simulink model "feedbackLin_Eq_Model"  (R2021a)
settings: Solver=ode1  StartTime=0.0  StopTime=150  FixedStep=0.005  RelTol=1e-3
undefined symbols (not defined in the file or in its folder): DiscIntNeverNeededParam
settings Model: Creator=laberobotica  LastModifiedBy=gabri

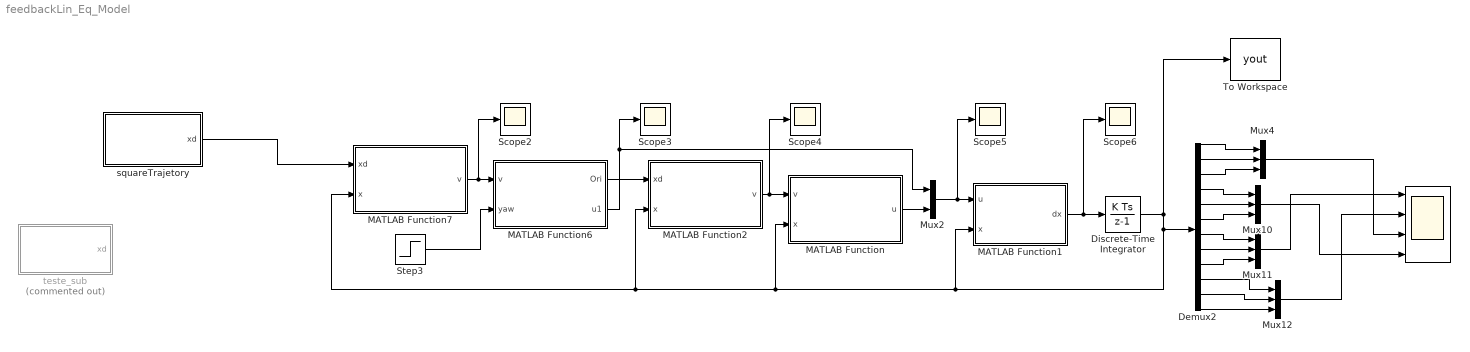
== system feedbackLin_Eq_Model ==
  " " : Scope  NumInputPorts=4
  Demux2 : Demux  Outputs=12
  Discrete-Time Integrator : DiscreteIntegrator  SampleTime=0.005  ICPrevOutput=DiscIntNeverNeededParam  ICPrevScaledInput=DiscIntNeverNeededParam
  MATLAB Function : MATLAB Function  TreatAsAtomicUnit=on
  MATLAB Function1 : MATLAB Function  TreatAsAtomicUnit=on
  MATLAB Function2 : MATLAB Function  TreatAsAtomicUnit=on
  MATLAB Function6 : MATLAB Function  TreatAsAtomicUnit=on
  MATLAB Function7 : MATLAB Function  TreatAsAtomicUnit=on
  Mux{4,10..12} (4 alike) : Mux  Inputs=3
  Mux2 : Mux  Inputs=2
  Scope{2..6} (5 alike) : Scope
  Step3 : Step  Time=35  After=0  SampleTime=0.005
  To Workspace : ToWorkspace  VariableName=yout  SampleTime=-1
      settings: Save2DSignal=2-D array (concatenate along first dimension)
  squareTrajetory : Subsystem
  teste_sub : Subsystem  Commented=on
  wires:
  MATLAB Function2/1(v) -> Scope4/1, MATLAB Function/1(v)
  MATLAB Function7/1(v) -> MATLAB Function6/1(v), Scope2/1
  Demux2/7 -> Mux11/1
  Demux2/9 -> Mux11/3
  Demux2/2 -> Mux4/2
  Demux2/10 -> Mux12/1
  Mux11/1 -> " "/1
  Mux4/1 -> " "/3
  Demux2/8 -> Mux11/2
  Discrete-Time Integrator/1 -> To Workspace/1, MATLAB Function1/2(x), MATLAB Function7/2(x), MATLAB Function2/2(x), MATLAB Function/2(x), Demux2/1
  Mux10/1 -> " "/4
  Mux12/1 -> " "/2
  Demux2/3 -> Mux4/3
  Demux2/11 -> Mux12/2
  Demux2/6 -> Mux10/3
  Demux2/12 -> Mux12/3
  Demux2/4 -> Mux10/1
  Demux2/5 -> Mux10/2
  Demux2/1 -> Mux4/1
  MATLAB Function6/2(u1) -> Mux2/1, Scope3/1
  MATLAB Function6/1(Ori) -> MATLAB Function2/1(xd)
  Step3/1 -> MATLAB Function6/2(yaw)
  MATLAB Function/1(u) -> Mux2/2
  Mux2/1 -> Scope5/1, MATLAB Function1/1(u)
  MATLAB Function1/1(dx) -> Discrete-Time Integrator/1, Scope6/1
  squareTrajetory/1(xd) -> MATLAB Function7/1(xd)

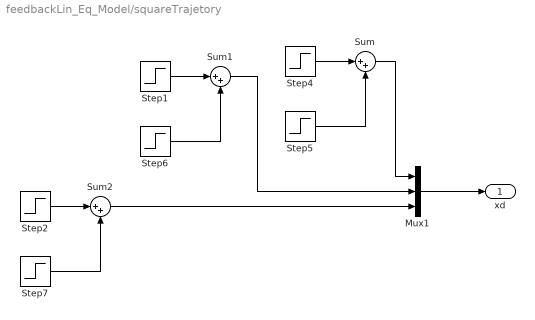
== system feedbackLin_Eq_Model/squareTrajetory ==
  Mux1 : Mux  Inputs=3
  Step1 : Step  Time=50  SampleTime=0.005
  Step2 : Step  Time=0  After=1.1  SampleTime=0.005
  Step4 : Step  Time=25  SampleTime=0.005
  Step5 : Step  Time=75  After=-1  SampleTime=0.005
  Step6 : Step  Time=100  After=-1  SampleTime=0.005
  Step7 : Step  Time=120  After=-1.1  SampleTime=0.005
  Sum : Sum  Inputs=|++
  Sum1 : Sum  Inputs=|++
  Sum2 : Sum  Inputs=|++
  xd : Outport
  wires:
  Step4/1 -> Sum/1
  Step1/1 -> Sum1/1
  Sum/1 -> Mux1/1
  Sum1/1 -> Mux1/2
  Step5/1 -> Sum/2
  Step7/1 -> Sum2/2
  Step6/1 -> Sum1/2
  Sum2/1 -> Mux1/3
  Step2/1 -> Sum2/1
  Mux1/1 -> xd/1

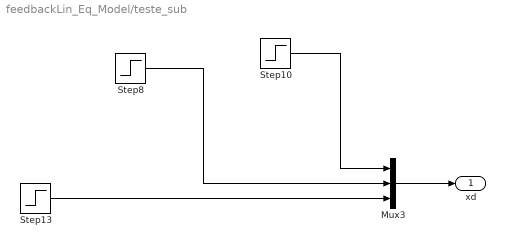
== system feedbackLin_Eq_Model/teste_sub ==
  Mux3 : Mux  Inputs=3
  Step10 : Step  Time=25  SampleTime=0.005
  Step13 : Step  Time=5  SampleTime=0.005
  Step8 : Step  Time=15  SampleTime=0.005
  xd : Outport
  wires:
  Mux3/1 -> xd/1
  Step8/1 -> Mux3/2
  Step10/1 -> Mux3/1
  Step13/1 -> Mux3/3

== matlab function feedbackLin_Eq_Model/MATLAB Function1 ==
  data: u input; dx output; x input
function dx  = DroneModel(u,x)

g = 9.81;
m = 0.063;
l = 0.0624*2;
Jx = 5.82857e-5;
Jy = 7.169148e-5;
Jz = 1e-4;

dx = zeros(1,12);

dx(1) = x(4);
dx(2) = x(5);
dx(3) = x(6);

dx(4) = -(cos(x(7)) * sin(x(8)) * cos(x(9)) + sin(x(7))*sin(x(9)))*(u(1)/m);

dx(5) = -(cos(x(7)) * sin(x(8)) * sin(x(9)) - sin(x(7))*cos(x(9)))*(u(1)/m);

dx(6) = g- (cos(x(7)) * cos(x(8)))*(u(1)/m);

dx(7) = x(10);
dx(8) = x(11);
dx(9) = x(12);

dx(10) = x(11)*x(12)*((Jy-Jz)/Jx)+(l/Jx)*u(2);
dx(11) = x(10)*x(12)*((Jz-Jx)/Jy)+(l/Jy)*u(3);
dx(12) = x(10)*x(11)*((Jx-Jy)/Jz)+(1/Jz)*u(4);
end

== matlab function feedbackLin_Eq_Model/MATLAB Function ==
  data: v input; u output; x input
function u = feedBackLinAtt(v, x)
g = 9.31;

m = 0.063;
l = 0.0624*2;
Jx = 5.82857e-5;
Jy = 7.169148e-5;
Jz = 1e-4;
K4 = -16; K3 = -16; K2 = -16;

u = zeros(1,3);

u(1) = (Jx/l)*(K2*x(10)-x(11)*x(12)*((Jy-Jz)/Jx))+v(1);
u(2) = (Jy/l)*(K3*x(11)-x(10)*x(12)*((Jz-Jx)/Jy))+v(2);
u(3) = (Jz)*(K4*x(12)-x(10)*x(11)*((Jx-Jy)/Jz))+v(3);
end

== matlab function feedbackLin_Eq_Model/MATLAB Function2 ==
  data: xd input; x input; v output
function v = ControlAttidude(xd,x)

w2 = 0.01; w3 = 0.01; w4 = 0.01;
v = zeros(1,3);

% controle de orientação
v(1) = w2*(xd(1) - x(7));
v(2) = w3*(xd(2) - x(8));
v(3) = w4*(xd(3) - x(9));


end

== matlab function feedbackLin_Eq_Model/MATLAB Function6 ==
  data: v input; Ori output; u1 output; yaw input
function [Ori,u1] = Calc_Ori(v,yaw)
g = 9.81;
m = 0.063;
l = 0.0624*2;
Jx = 5.82857e-5;
Jy = 7.169148e-5;
Jz = 1e-4;
Ori = zeros(1,3);
u1=0;

u1 = m*((v(1)^2)+(v(2)^2)+((g-v(3))^2))^0.5;  %m*sqrt(((v(1)/beta)^2)+v(2)^2)

beta = (v(1)/u1)*m;

alpha = (v(2)/u1)*m;

Ori(1)=asin(alpha);
Ori(2)=-asin(beta);
Ori(3) = yaw;


end

== matlab function feedbackLin_Eq_Model/MATLAB Function7 ==
  data: xd input; x input; v output
function v = ControlAlt(xd,x)

k1 = 0.22; k2=0.22; k3=0.22;
v = zeros(1,3);


v(1) = k1*(xd(1) - x(1))+(-0.8*x(4));%
v(2) = k2*(xd(2) - x(2))+(-0.8*x(5));
v(3) = k3*(xd(3) - x(3))+(-0.8*x(6));

end
